simulink library "ErrorCodeGenerator"  (R2016b)
settings: Solver=VariableStepAuto  StartTime=0.0  StopTime=10.0  RelTol=1e-3
settings Model: Creator=Nathan  LastModifiedBy=Marc

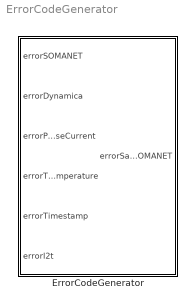
== system ErrorCodeGenerator ==
  ErrorCodeGenerator : Subsystem

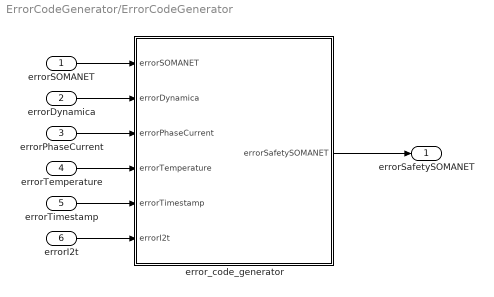
== system ErrorCodeGenerator/ErrorCodeGenerator ==
  errorSOMANET : Inport
  errorDynamica : Inport  Port=2
  errorPhaseCurrent : Inport  Port=3
  errorTemperature : Inport  Port=4
  errorTimestamp : Inport  Port=5
  errorI2t : Inport  Port=6
  error_code_generator : MATLAB Function  TreatAsAtomicUnit=on
  errorSafetySOMANET : Outport
  wires:
  errorSOMANET/1 -> error_code_generator/1(errorSOMANET)
  errorTimestamp/1 -> error_code_generator/5(errorTimestamp)
  errorDynamica/1 -> error_code_generator/2(errorDynamica)
  errorPhaseCurrent/1 -> error_code_generator/3(errorPhaseCurrent)
  errorTemperature/1 -> error_code_generator/4(errorTemperature)
  error_code_generator/1(errorSafetySOMANET) -> errorSafetySOMANET/1
  errorI2t/1 -> error_code_generator/6(errorI2t)

== matlab function ErrorCodeGenerator/error_code_generator ==
  data: errorSOMANET input; errorDynamica input; errorSafetySOMANET output; errorPhaseCurrent input; errorTemperature input; errorTimestamp input; errorI2t input
function errorSafetySOMANET = error_code_generator(errorSOMANET,errorDynamica,errorPhaseCurrent,errorTemperature,errorTimestamp, errorI2t)
persistent error;

if(isempty(error))
    error = 0;
end
%% errorI2t
%   1: integral of current^2 exceeded the maximum
%   (=curentTimeMaximum*(currentMaximum^2 - currentNominal^2))
error = error + bitshift(errorI2t, 5);
%% errorDynamica 
%   1: angle does or will exceed soft stops
%   2: velocity does or will exceed the maximum allowed velocity
%   3: the torque does or will exceed the maximum allowed torque
%   4: the difference between the actual angle and the target angle is too big
%   5: the difference between the actual velocity and the target velocity is  too big
error = error + bitshift(errorDynamica,4);
%% errorPhaseCurrent
%   1: the phase current does exceed the maximum allowed current
error = error + bitshift(errorPhaseCurrent,3);
%% errorTemperature
%   1: the measured temperature does exceed the maximum allowed temperature
error = error + bitshift(errorTemperature,2);
%% errorTimestamp
%   1: the SOMANET has responded for longer than the maximum allowed non responsive time.
error = error + bitshift(errorTimestamp,1);
%% errorSOMANET
% If error occurs in SOMANET, let it have influence on the error
error = error + bitshift(errorSOMANET,0);

errorSafetySOMANET = error;
